simulink model "AsynchronousExample"  (R2023a)
settings: Solver=VariableStepAuto  StartTime=0.0  StopTime=10.0  RelTol=1e-3
settings Model: Creator=Administrator  LastModifiedBy=wkmiao
settings RTWCC: GPUComputeCapability=5.0

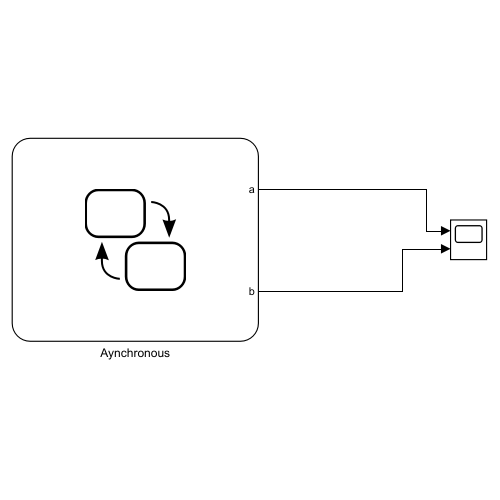
[thumbnail: Simulink's stored preview of the top-level diagram]
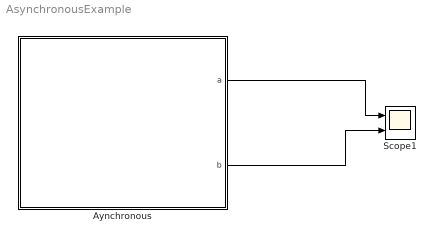
== system AsynchronousExample ==
  Aynchronous : Stateflow chart  TreatAsAtomicUnit=on
  Scope1 : Scope  NumInputPorts=2
  wires:
  Aynchronous/1(a) -> Scope1/1
  Aynchronous/2(b) -> Scope1/2

== stateflow chart AsynchronousExample/Aynchronous ==
  settings: initializeOutput=1
  state outputa [parallel]
    settings: executionOrder=1
    state s1
    state s2
    (default) -> s1
    s1 -> s2 : [rand()>0.5]{a = 1}
    s2 -> s1 : [rand()>0.5]{a=0}
  state outputb [parallel]
    settings: executionOrder=2
    state s3
    state s4
    (default) -> s3
    s3 -> s4 : [rand()>0.8]{b=0}
    s4 -> s3 : [rand()>0.65]{b = 2}
  data: a output; b output
